simulink model "gm_BlobAnalysisHDL"  (R2022b)
settings: Solver=FixedStepDiscrete  StartTime=0.0  StopTime=1/60  RelTol=1e-3
PreLoadFcn:
  | model_init_cca
InitFcn:
  | model_init_cca
undefined symbols (not defined in the file or in its folder): closenhood, gray, MaxBlobs, numCols, numRows, Rec, rgbmap24, SDTV, Ts
libraries: hdlsllib x37, simulink x21, hdlmdlgenlib x7, visionhdlutilities x5, visionhdlio x2, visiontextngfix x2, visionhdlmorphops x1, visionhdlconversions x1, visionsources x1, visiongeotforms x1
(part 1 of 3)
settings Model: SimulationMode=accelerator  Creator=The MathWorks, Inc.  LastModifiedBy=team06
settings SolverCC: AlgebraicLoopSolver=TrustRegion
settings DataIOCC: SaveOutput=off  SaveTime=off
settings OptimizationCC: BlockReduction=off  ConditionallyExecuteInputs=off  DefaultParameterBehavior=Inlined
settings DebuggingCC: AlgebraicLoopMsg=error  InheritedTsInSrcMsg=none  SingleTaskRateTransMsg=error  ParameterDowncastMsg=none  ParameterOverflowMsg=none  UnconnectedInputMsg=warning  UnconnectedOutputMsg=warning  UnconnectedLineMsg=warning  SFMachineParentedDataDiag=warning
settings HardwareCC: ProdBitPerPointer=32  ProdBitPerSizeT=32  ProdBitPerPtrDiffT=32  ProdLargestAtomicFloat=None  ProdIntDivRoundTo=Undefined  ProdEndianess=Unspecified  ProdWordSize=32  ProdHWDeviceType=ASIC/FPGA->ASIC/FPGA  TargetBitPerPointer=64  TargetBitPerSizeT=64  TargetBitPerPtrDiffT=64  TargetLongLongMode=on  TargetIntDivRoundTo=Zero  TargetEndianess=LittleEndian  TargetWordSize=64  TargetHWDeviceType=Custom Processor->MATLAB Host Computer  ProdEqTarget=off
settings ModelReferenceCC: EnableRefExpFcnMdlSchedulingChecks=on
settings RTWCC: DLArmComputeVersion=19.05

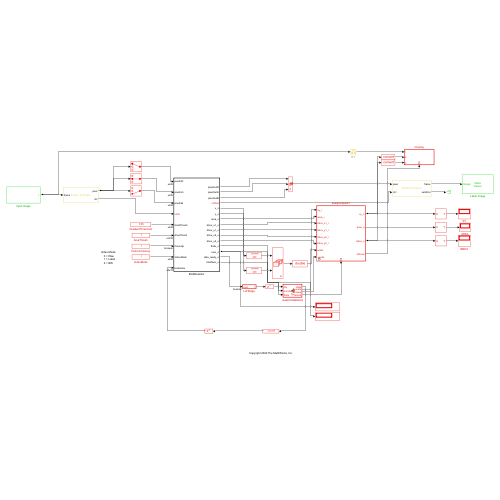
[thumbnail: Simulink's stored preview of the top-level diagram]
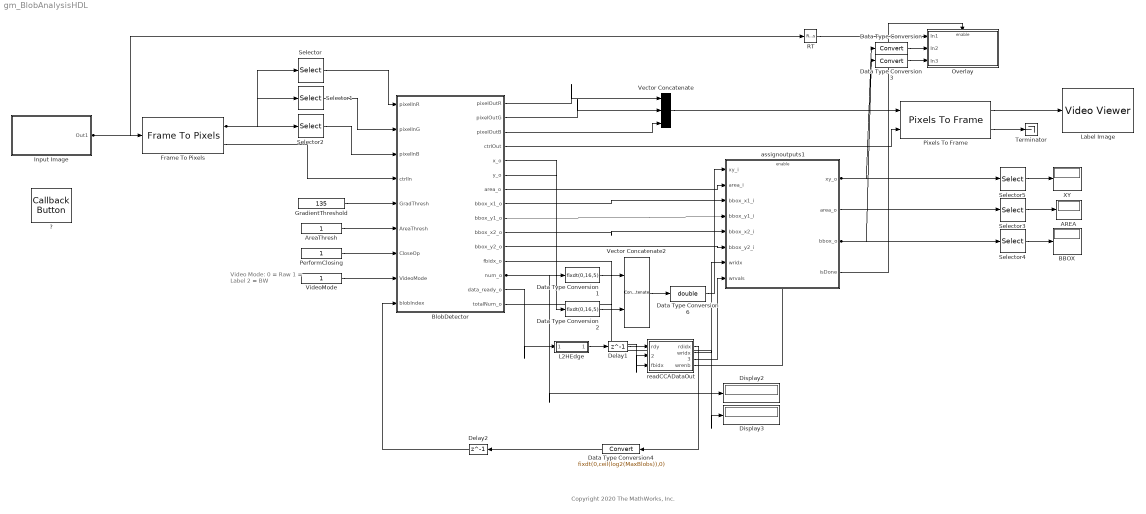
== system gm_BlobAnalysisHDL ==
  note: Copyright 2020 The MathWorks, Inc.
  note: Video Mode:
      |     0 = Raw
      |     1 = Label
      |     2 = BW
  "?" : CallbackButton  ButtonText=?
      settings: ClickFcn=showExample('visionhdl/BlobAnalysisExample')
  AREA : Display
  AreaThresh : Constant  OutDataTypeStr=uint32  SampleTime=-1
  BBOX : Display
  BlobDetector : Subsystem  TreatAsAtomicUnit=on
  Data Type Conversion : DataTypeConversion  SaturateOnIntegerOverflow=off  RndMeth=Floor
  Data Type Conversion1 : DataTypeConversion  OutDataTypeStr=fixdt(0,16,5)  ConvertRealWorld=Stored Integer (SI)  SaturateOnIntegerOverflow=off  RndMeth=Floor
  Data Type Conversion2 : DataTypeConversion  OutDataTypeStr=fixdt(0,16,5)  ConvertRealWorld=Stored Integer (SI)  SaturateOnIntegerOverflow=off  RndMeth=Floor
  Data Type Conversion3 : DataTypeConversion  SaturateOnIntegerOverflow=off  RndMeth=Floor
  Data Type Conversion4 : DataTypeConversion  OutDataTypeStr=fixdt(0,ceil(log2(MaxBlobs)),0)  SaturateOnIntegerOverflow=off  RndMeth=Floor
  Data Type Conversion6 : DataTypeConversion  OutDataTypeStr=double  SaturateOnIntegerOverflow=off  RndMeth=Floor
  Delay1 : Delay  DelayLength=1
  Delay2 : Delay  DelayLength=1
  Display2 : Display
  Display3 : Display
  Frame To Pixels : visionhdlio/Frame To Pixels  NumComponents=3  NumPixels=1  VideoFormat=240p  ActivePixelsPerLine=320  ActiveVideoLines=240  TotalPixelsPerLine=402  TotalVideoLines=324  StartingActiveLine=1  FrontPorch=44  SampleTime=0  VideoFormatCache=240p  ActivePixelsPerLineCache=numCols  ActiveVideoLinesCache=numRows  TotalPixelsPerLineCache=numCols+50  TotalVideoLinesCache=numRows+5  StartingActiveLineCache=2  FrontPorchCache=2
  GradientThreshold : Constant  Value=135  OutDataTypeStr=uint8  SampleTime=-1
  Input Image : Subsystem
  L2HEdge : Subsystem  TreatAsAtomicUnit=on
  Label Image : VideoViewer  FigPos=[539 508 418 304]
  Overlay : Subsystem
  PerformClosing : Constant  OutDataTypeStr=boolean  SampleTime=-1
  Pixels To Frame : visionhdlio/Pixels To Frame  NumComponents=3  NumPixels=1  VideoFormat=240p  ActivePixelsPerLine=320  ActiveVideoLines=240  TotalPixelsPerLine=402  TotalVideoLines=324  VideoFormatCache=240p  ActivePixelsPerLineCache=numCols  ActiveVideoLinesCache=numRows  TotalPixelsPerLineCache=numCols+50  TotalVideoLinesCache=numRows+5
  RT : RateTransition  Deterministic=off  OutPortSampleTimeOpt=Inherit  OutPortSampleTime=1.2796101795549e-07
  Selector : Selector  InputPortWidth=3  IndexOptions=Index vector (dialog)  Indices=1  OutputSizes=1
  Selector1 : Selector  InputPortWidth=3  IndexOptions=Index vector (dialog)  Indices=2  OutputSizes=1
  Selector2 : Selector  InputPortWidth=3  IndexOptions=Index vector (dialog)  Indices=3  OutputSizes=1
  Selector3 : Selector  NumberOfDimensions=2  InputPortWidth=3  IndexOptions=Index vector (dialog),Select all  Indices=1:20,1:200  OutputSizes=1,1
  Selector4 : Selector  NumberOfDimensions=2  InputPortWidth=3  IndexOptions=Index vector (dialog),Select all  Indices=1:20,1:200  OutputSizes=1,1
  Selector5 : Selector  NumberOfDimensions=2  InputPortWidth=3  IndexOptions=Index vector (dialog),Select all  Indices=1:20,1:200  OutputSizes=1,1
  Terminator : Terminator
  Vector Concatenate : Concatenate  NumInputs=3  Mode=Multidimensional array  ConcatenateDimension=2
  Vector Concatenate2 : Concatenate  Mode=Multidimensional array  ConcatenateDimension=2
  VideoMode : Constant  OutDataTypeStr=uint8  SampleTime=-1
  XY : Display
  assignoutputs1 : Subsystem
  readCCADataOut : MATLAB Function  TreatAsAtomicUnit=on  mask{maxnumblobs=MaxBlobs}
      mask prompts: maxnumblobs "Max number of blobs"
  wires:
  Selector5/1 -> XY/1
  Selector4/1 -> BBOX/1
  Selector3/1 -> AREA/1
  Input Image/1(Out1) -> Frame To Pixels/1, RT/1
  Frame To Pixels/1 -> Selector2/1, Selector/1, Selector1/1
  Selector1/1 -> BlobDetector/2(pixelInG)
  readCCADataOut/3(wrvalue) -> assignoutputs1/8(wrvals)
  Data Type Conversion4/1 -> Delay2/1
  Vector Concatenate/1 -> Pixels To Frame/1
  BlobDetector/8(bbox_x1_o) -> assignoutputs1/3(bbox_x1_i)
  RT/1 -> Overlay/1(In1)
  readCCADataOut/2(wridx) -> assignoutputs1/7(wridx)
  L2HEdge/1(Out1) -> Delay1/1
  Vector Concatenate2/1 -> Data Type Conversion6/1
  assignoutputs1/1(xy_o) -> Data Type Conversion/1, Selector5/1
  BlobDetector/10(bbox_x2_o) -> assignoutputs1/5(bbox_x2_i)
  GradientThreshold/1 -> BlobDetector/5(GradThresh)
  Data Type Conversion2/1 -> Vector Concatenate2/2
  Data Type Conversion3/1 -> Overlay/3(In3)
  VideoMode/1 -> BlobDetector/8(VideoMode)
  AreaThresh/1 -> BlobDetector/6(AreaThresh)
  BlobDetector/4(ctrlOut) -> Pixels To Frame/2
  assignoutputs1/4(isDone) -> Overlay/Enable
  Data Type Conversion6/1 -> assignoutputs1/1(xy_i)
  Selector2/1 -> BlobDetector/3(pixelInB)
  PerformClosing/1 -> BlobDetector/7(CloseOp)
  Delay1/1 -> readCCADataOut/1(rdy)
  Frame To Pixels/2 -> BlobDetector/4(ctrlIn)
  BlobDetector/6(y_o) -> Data Type Conversion2/1
  BlobDetector/9(bbox_y1_o) -> assignoutputs1/4(bbox_y1_i)
  BlobDetector/13(num_o) -> Display2/1, readCCADataOut/2(num2rd)
  Pixels To Frame/2 -> Terminator/1
  readCCADataOut/4(wrenb) -> assignoutputs1/Enable
  BlobDetector/12(fbidx_o) -> readCCADataOut/3(fbidx)
  Data Type Conversion1/1 -> Vector Concatenate2/1
  Delay2/1 -> BlobDetector/9(blobIndex)
  Selector/1 -> BlobDetector/1(pixelInR)
  BlobDetector/2(pixelOutG) -> Vector Concatenate/2
  assignoutputs1/2(area_o) -> Selector3/1
  BlobDetector/3(pixelOutB) -> Vector Concatenate/3
  BlobDetector/7(area_o) -> assignoutputs1/2(area_i)
  BlobDetector/11(bbox_y2_o) -> assignoutputs1/6(bbox_y2_i)
  readCCADataOut/1(rdidx) -> Data Type Conversion4/1
  assignoutputs1/3(bbox_o) -> Data Type Conversion3/1, Selector4/1
  BlobDetector/5(x_o) -> Data Type Conversion1/1
  BlobDetector/14(data_ready_o) -> L2HEdge/1(sync)
  Pixels To Frame/1 -> Label Image/1
  Data Type Conversion/1 -> Overlay/2(In2)
  BlobDetector/15(totalNum_o) -> Display3/1
  BlobDetector/1(pixelOutR) -> Vector Concatenate/1

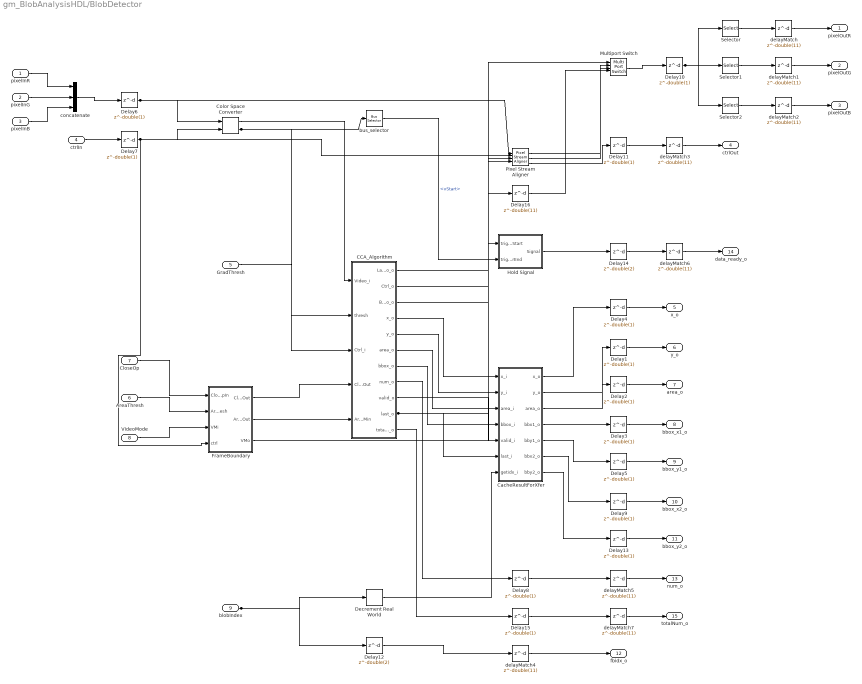
== system gm_BlobAnalysisHDL/BlobDetector ==
  pixelInR : Inport  OutDataTypeStr=uint8  PortDimensions=1  SampleTime=1.2796101795549e-07
  pixelInG : Inport  Port=2  OutDataTypeStr=uint8  PortDimensions=1  SampleTime=1.2796101795549e-07
  pixelInB : Inport  Port=3  OutDataTypeStr=uint8  PortDimensions=1  SampleTime=1.2796101795549e-07
  ctrlIn : Inport  Port=4
  GradThresh : Inport  Port=5  OutDataTypeStr=uint8  PortDimensions=1  SampleTime=1.2796101795549e-07
  AreaThresh : Inport  Port=6  OutDataTypeStr=uint32  PortDimensions=1  SampleTime=1.2796101795549e-07
  CloseOp : Inport  Port=7  OutDataTypeStr=boolean  PortDimensions=1  SampleTime=1.2796101795549e-07
  VideoMode : Inport  Port=8  OutDataTypeStr=uint8  PortDimensions=1  SampleTime=1.2796101795549e-07
  blobIndex : Inport  Port=9  OutDataTypeStr=fixdt(0, 10, 0)  PortDimensions=1  SampleTime=1.2796101795549e-07
  CCA_Algorithm : Subsystem
  CacheResultForXfer : Subsystem
  Color Space Converter : visionhdlconversions/Color Space Converter  Conversion=RGB to intensity  ConversionStandard=Rec. 601 (SDTV)  ScanningStandard=1250/50/2:1  SimulateUsing=Code generation
  Decrement Real World : simulink/Additional Math & Discrete/Additional Math: Increment - Decrement/Decrement Real World
  Delay{1..6,8..10,13,15} (11 alike) : Delay  DelayLength=double(1)  InitialCondition=0  SampleTime=1.2796101795549e-07
  Delay11 : Delay  DelayLength=double(1)  SampleTime=1.2796101795549e-07
  Delay12 : Delay  DelayLength=double(2)  InitialCondition=0  SampleTime=1.2796101795549e-07
  Delay14 : Delay  DelayLength=double(2)  InitialCondition=0  SampleTime=1.2796101795549e-07
  Delay16 : Delay  DelayLength=double(11)  InitialCondition=0  SampleTime=1.2796101795549e-07
  Delay7 : Delay  DelayLength=double(1)  SampleTime=1.2796101795549e-07
  FrameBoundary : Subsystem
  Hold Signal : Subsystem
  Multiport Switch : MultiPortSwitch  DataPortOrder=Zero-based contiguous  DiagnosticForDefault=None  zeroidx=on  OutDataTypeStr=uint8  SampleTime=1.2796101795549e-07  SaturateOnIntegerOverflow=off  InputSameDT=off
  Pixel Stream Aligner : visionhdlutilities/Pixel Stream Aligner  LineBufferSize=2048  MaximumNumberOfLines=size(closenhood.Neighborhood,1)+1  SimulateUsing=Code generation
  Selector : Selector  SampleTime=1.2796101795549e-07  IndexOptions=Index vector (dialog)  Indices=double(1)  OutputSizes=double(1)
  Selector1 : Selector  SampleTime=1.2796101795549e-07  IndexOptions=Index vector (dialog)  Indices=double(2)  OutputSizes=double(1)
  Selector2 : Selector  SampleTime=1.2796101795549e-07  IndexOptions=Index vector (dialog)  Indices=double(3)  OutputSizes=double(1)
  bus_selector : BusSelector  OutputSignals=vStart
  concatenate : Concatenate  NumInputs=3  Mode=Multidimensional array  ConcatenateDimension=2
  delayMatch{,1..7} (8 alike) : Delay  DelayLength=double(11)  InitialCondition=0  SampleTime=1.2796101795549e-07
  pixelOutR : Outport  SampleTime=1.2796101795549e-07  VectorParamsAs1DForOutWhenUnconnected=off
  pixelOutG : Outport  Port=2  SampleTime=1.2796101795549e-07  VectorParamsAs1DForOutWhenUnconnected=off
  pixelOutB : Outport  Port=3  SampleTime=1.2796101795549e-07  VectorParamsAs1DForOutWhenUnconnected=off
  ctrlOut : Outport  Port=4  VectorParamsAs1DForOutWhenUnconnected=off
  x_o : Outport  Port=5  SampleTime=1.2796101795549e-07  VectorParamsAs1DForOutWhenUnconnected=off
  y_o : Outport  Port=6  SampleTime=1.2796101795549e-07  VectorParamsAs1DForOutWhenUnconnected=off
  area_o : Outport  Port=7  SampleTime=1.2796101795549e-07  VectorParamsAs1DForOutWhenUnconnected=off
  bbox_x1_o : Outport  Port=8  SampleTime=1.2796101795549e-07  VectorParamsAs1DForOutWhenUnconnected=off
  bbox_y1_o : Outport  Port=9  SampleTime=1.2796101795549e-07  VectorParamsAs1DForOutWhenUnconnected=off
  bbox_x2_o : Outport  Port=10  SampleTime=1.2796101795549e-07  VectorParamsAs1DForOutWhenUnconnected=off
  bbox_y2_o : Outport  Port=11  SampleTime=1.2796101795549e-07  VectorParamsAs1DForOutWhenUnconnected=off
  fbidx_o : Outport  Port=12  SampleTime=1.2796101795549e-07  VectorParamsAs1DForOutWhenUnconnected=off
  num_o : Outport  Port=13  SampleTime=1.2796101795549e-07  VectorParamsAs1DForOutWhenUnconnected=off
  data_ready_o : Outport  Port=14  SampleTime=1.2796101795549e-07  VectorParamsAs1DForOutWhenUnconnected=off
  totalNum_o : Outport  Port=15  SampleTime=1.2796101795549e-07  VectorParamsAs1DForOutWhenUnconnected=off
  wires:
  pixelInR/1 -> concatenate/1
  pixelInG/1 -> concatenate/2
  pixelInB/1 -> concatenate/3
  ctrlIn/1 -> Delay7/1
  GradThresh/1 -> CCA_Algorithm/2(thresh)
  AreaThresh/1 -> FrameBoundary/2(AreaThresh)
  CloseOp/1 -> FrameBoundary/1(CloseOpIn)
  VideoMode/1 -> FrameBoundary/3(VMi)
  blobIndex/1 -> Decrement Real World/1, Delay12/1
  bus_selector/1 -> Hold Signal/2(triggerEnd)  "<vStart>"
  CCA_Algorithm/1(LabelVideo_o) -> Pixel Stream Aligner/3
  CCA_Algorithm/2(Ctrl_o) -> Pixel Stream Aligner/4
  CCA_Algorithm/3(BWVideo_o) -> Delay16/1
  CCA_Algorithm/4(x_o) -> CacheResultForXfer/1(x_i)
  CCA_Algorithm/5(y_o) -> CacheResultForXfer/2(y_i)
  CCA_Algorithm/6(area_o) -> CacheResultForXfer/3(area_i)
  CCA_Algorithm/7(bbox_o) -> CacheResultForXfer/4(bbox_i)
  CCA_Algorithm/8(num_o) -> Delay8/1
  CCA_Algorithm/9(valid_o) -> CacheResultForXfer/5(valid_i)
  CCA_Algorithm/10(last_o) -> Hold Signal/1(triggerStart), CacheResultForXfer/6(last_i)
  CCA_Algorithm/11(totalNum_o) -> Delay15/1
  CacheResultForXfer/1(x_o) -> Delay4/1
  CacheResultForXfer/2(y_o) -> Delay1/1
  CacheResultForXfer/3(area_o) -> Delay2/1
  CacheResultForXfer/4(bbx1_o) -> Delay3/1
  CacheResultForXfer/5(bby1_o) -> Delay5/1
  CacheResultForXfer/6(bbx2_o) -> Delay9/1
  CacheResultForXfer/7(bby2_o) -> Delay13/1
  Color Space Converter/1 -> CCA_Algorithm/1(Video_i)
  Color Space Converter/2 -> bus_selector/1, CCA_Algorithm/3(Ctrl_i)
  Decrement Real World/1 -> CacheResultForXfer/7(getidx_i)
  Delay1/1 -> y_o/1
  Delay10/1 -> Selector2/1, Selector1/1, Selector/1
  delayMatch3/1 -> ctrlOut/1
  delayMatch4/1 -> fbidx_o/1
  Delay13/1 -> bbox_y2_o/1
  delayMatch6/1 -> data_ready_o/1
  delayMatch7/1 -> totalNum_o/1
  Delay16/1 -> Multiport Switch/4
  Delay2/1 -> area_o/1
  Delay3/1 -> bbox_x1_o/1
  Delay4/1 -> x_o/1
  Delay5/1 -> bbox_y1_o/1
  Delay6/1 -> Pixel Stream Aligner/1, Color Space Converter/1
  Delay7/1 -> FrameBoundary/4(ctrl), Pixel Stream Aligner/2, Color Space Converter/2
  delayMatch5/1 -> num_o/1
  Delay9/1 -> bbox_x2_o/1
  FrameBoundary/1(CloseOpOut) -> CCA_Algorithm/4(CloseOpOut)
  FrameBoundary/2(AreaThreshOut) -> CCA_Algorithm/5(AreaMin)
  FrameBoundary/3(VMo) -> Multiport Switch/1
  Hold Signal/1(Signal) -> Delay14/1
  Multiport Switch/1 -> Delay10/1
  Pixel Stream Aligner/1 -> Multiport Switch/2
  Pixel Stream Aligner/2 -> Multiport Switch/3
  Pixel Stream Aligner/3 -> Delay11/1
  delayMatch/1 -> pixelOutR/1
  delayMatch1/1 -> pixelOutG/1
  delayMatch2/1 -> pixelOutB/1
  concatenate/1 -> Delay6/1
  Selector/1 -> delayMatch/1
  Selector1/1 -> delayMatch1/1
  Selector2/1 -> delayMatch2/1
  Delay11/1 -> delayMatch3/1
  Delay12/1 -> delayMatch4/1
  Delay8/1 -> delayMatch5/1
  Delay14/1 -> delayMatch6/1
  Delay15/1 -> delayMatch7/1

== system gm_BlobAnalysisHDL/Input Image ==
  Constant : Constant  Value=true  VectorParams1D=off  SampleTime=-1
  Data Type Conversion : DataTypeConversion  OutDataTypeStr=uint8  SaturateOnIntegerOverflow=off  RndMeth=Floor
  Delay : Delay  DelayLength=1  InitialCondition=0  UseCircularBuffer=on
  Delay1 : Delay  DelayLength=1  InitialCondition=0  ShowEnablePort=on  UseCircularBuffer=on
      settings: InputPortMap=u0,e6
  Image From File : visionsources/Image From File  Tag=vipblks_nd  FileName=coins.png  Ts=1/60  imagePorts=One multidimensional signal  OutPortLabels=R|G|B  ImageDataType=Inherit from input image  sdImageDataType=uint(8)  Signed=on  WordLength=16  FractionLengthMode=User-defined  FractionLength=15
  Matrix Concatenate : Concatenate  NumInputs=3  Mode=Multidimensional array  ConcatenateDimension=3
  Matrix Concatenate1 : Concatenate  Mode=Multidimensional array  ConcatenateDimension=2
  Multiport Switch : MultiPortSwitch  DataPortOrder=Zero-based contiguous  Inputs=2  zeroidx=on  SaturateOnIntegerOverflow=off  InputSameDT=off
  Resize : visiongeotforms/Resize  specify=Number of output rows and columns  rfactor=[200 150]  outCols=25  outRows=25  outRowsCols=[240 320]  interp_method=Bilinear  antialias=on  useROI=off  roiFlag=off  roundingMode=Nearest  overflowMode=on  prodOutputMode=Binary point scaling  prodOutputWordLength=32  prodOutputFracLength=10
  Selector : Selector  NumberOfDimensions=2  InputPortWidth=3  IndexOptions=Select all,Index vector (dialog)  Indices=[1 3],301:320  OutputSizes=1,1
  Selector1 : Selector  NumberOfDimensions=2  InputPortWidth=3  IndexOptions=Select all,Index vector (dialog)  Indices=[1 3],1:300  OutputSizes=1,1
  Out1 : Outport
  wires:
  Data Type Conversion/1 -> Out1/1
  Delay1/1 -> Multiport Switch/1
  Constant/1 -> Delay1/1, Delay1/2
  Delay/1 -> Multiport Switch/3
  Selector1/1 -> Matrix Concatenate1/2
  Selector/1 -> Matrix Concatenate1/1
  Multiport Switch/1 -> Selector/1, Selector1/1, Matrix Concatenate/1, Matrix Concatenate/2, Matrix Concatenate/3
  Matrix Concatenate1/1 -> Delay/1
  Resize/1 -> Multiport Switch/2
  Image From File/1 -> Resize/1
  Matrix Concatenate/1 -> Data Type Conversion/1

== system gm_BlobAnalysisHDL/L2HEdge ==
  sync : Inport  OutDataTypeStr=boolean
  Logical Operator : Logic  Operator=XOR  IconShape=distinctive  AllPortsSameDT=off  OutDataTypeStr=boolean
  Logical Operator2 : Logic  IconShape=distinctive  AllPortsSameDT=off  OutDataTypeStr=boolean
  Unit Delay : UnitDelay  SampleTime=-1  HasFrameUpgradeWarning=on
  Out1 : Outport  VectorParamsAs1DForOutWhenUnconnected=off
  wires:
  Logical Operator2/1 -> Out1/1
  Logical Operator/1 -> Logical Operator2/1
  Unit Delay/1 -> Logical Operator/1
  sync/1 -> Logical Operator2/2, Logical Operator/2, Unit Delay/1

== system gm_BlobAnalysisHDL/Overlay ==
  In1 : Inport
  In2 : Inport  Port=2
  In3 : Inport  Port=3
  Enable : EnablePort
  Draw Markers : visiontextngfix/Draw Markers  shape=Plus  size=1  fill=on  fillClrSource=Specify via dialog  display=User-specified value  intensity=200  color=[255 20 20]  opacity=1  viewport=Entire image  antialiasing=off  inType=Obsolete  imagePorts=One multidimensional signal  roundingMode=Floor  overflowMode=off  memoryMode=Specify word length  memoryWordLength=16  memoryFracLength=15  prodOutputMode=Binary point scaling  prodOutputWordLength=32  prodOutputFracLength=14
  Draw Shapes : visiontextngfix/Draw Shapes  shape=Rectangles  fill=off  lineWidth=1  fillClrSource=Specify via dialog  display=User-specified value  intensity=200  color=[20 255 10]  opacity=0.6  viewport=Entire image  antialiasing=off  inType=Obsolete  imagePorts=One multidimensional signal  roundingMode=Floor  overflowMode=off  memoryMode=Specify word length  memoryWordLength=16  prodOutputMode=Binary point scaling  prodOutputWordLength=32  prodOutputFracLength=14  memoryFracLength=15
  Results On Image : VideoViewer  colormapValue=gray(256)  FigPos=[117 509 417 304]
  wires:
  Draw Markers/1 -> Draw Shapes/1
  In3/1 -> Draw Shapes/2
  In2/1 -> Draw Markers/2
  In1/1 -> Draw Markers/1
  Draw Shapes/1 -> Results On Image/1

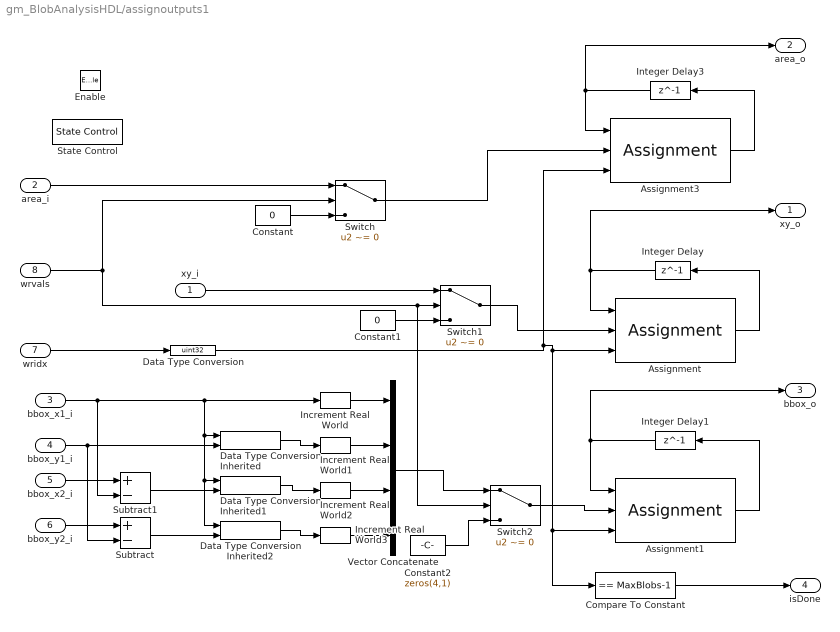
== system gm_BlobAnalysisHDL/assignoutputs1 ==
  xy_i : Inport
  area_i : Inport  Port=2
  bbox_x1_i : Inport  Port=3
  bbox_y1_i : Inport  Port=4
  bbox_x2_i : Inport  Port=5
  bbox_y2_i : Inport  Port=6
  wridx : Inport  Port=7
  wrvals : Inport  Port=8
  Enable : EnablePort
  Assignment : Assignment  NumberOfDimensions=2  DiagnosticForDimensions=Warning  IndexOptions=Starting index (port),Assign all  Indices=1,1  OutputSizes=1,1
  Assignment1 : Assignment  NumberOfDimensions=2  DiagnosticForDimensions=Warning  IndexOptions=Starting index (port),Assign all  Indices=1,1  OutputSizes=1,1
  Assignment3 : Assignment  NumberOfDimensions=2  DiagnosticForDimensions=Warning  IndexOptions=Starting index (port),Assign all  Indices=1,1  OutputSizes=1,1
  Compare To Constant : simulink/Logic and Bit Operations/Compare To Constant  relop===  const=MaxBlobs-1  OutDataTypeStr=boolean
  Constant : Constant  Value=0  OutDataTypeStr=Inherit: Inherit via back propagation  SampleTime=-1
  Constant1 : Constant  Value=0  OutDataTypeStr=Inherit: Inherit via back propagation  SampleTime=-1
  Constant2 : Constant  Value=zeros(4,1)  OutDataTypeStr=Inherit: Inherit via back propagation  SampleTime=-1
  Data Type Conversion Inherited : simulink/Signal Attributes/Data Type Conversion Inherited  ConvertRealWorld=Real World Value  DoSatur=off
  Data Type Conversion Inherited1 : simulink/Signal Attributes/Data Type Conversion Inherited  ConvertRealWorld=Real World Value  DoSatur=off
  Data Type Conversion Inherited2 : simulink/Signal Attributes/Data Type Conversion Inherited  ConvertRealWorld=Real World Value  DoSatur=off
  Data Type Conversion : DataTypeConversion  OutDataTypeStr=uint32  SaturateOnIntegerOverflow=off  RndMeth=Floor
  Increment Real World{,1..3} (4 alike) : simulink/Additional Math & Discrete/Additional Math: Increment - Decrement/Increment Real World
  Integer Delay : Delay  DelayLength=1  InitialCondition=zeros(MaxBlobs,2)
  Integer Delay1 : Delay  DelayLength=1  InitialCondition=zeros(MaxBlobs,4)
  Integer Delay3 : Delay  DelayLength=1  InitialCondition=zeros(MaxBlobs,1)
  State Control : StateControl  StateControl=Synchronous
  Subtract : Sum  Inputs=+-  OutDataTypeStr=Inherit: Same as first input
  Subtract1 : Sum  Inputs=+-  OutDataTypeStr=Inherit: Same as first input
  Switch : Switch  Criteria=u2 ~= 0  SaturateOnIntegerOverflow=off  InputSameDT=off
  Switch1 : Switch  Criteria=u2 ~= 0  SaturateOnIntegerOverflow=off  InputSameDT=off
  Switch2 : Switch  Criteria=u2 ~= 0  SaturateOnIntegerOverflow=off  InputSameDT=off
  Vector Concatenate : Concatenate  NumInputs=4  Mode=Multidimensional array  ConcatenateDimension=2
  xy_o : Outport  VectorParamsAs1DForOutWhenUnconnected=off
  area_o : Outport  Port=2  VectorParamsAs1DForOutWhenUnconnected=off
  bbox_o : Outport  Port=3  VectorParamsAs1DForOutWhenUnconnected=off
  isDone : Outport  Port=4  VectorParamsAs1DForOutWhenUnconnected=off
  wires:
  wridx/1 -> Data Type Conversion/1
  Compare To Constant/1 -> isDone/1
  Data Type Conversion/1 -> Assignment1/3, Compare To Constant/1, Assignment/3, Assignment3/3
  Switch2/1 -> Assignment1/2
  Constant2/1 -> Switch2/3
  xy_i/1 -> Switch1/1
  Constant1/1 -> Switch1/3
  Switch/1 -> Assignment3/2
  Constant/1 -> Switch/3
  area_i/1 -> Switch/1
  wrvals/1 -> Switch/2, Switch1/2, Switch2/2
  Assignment/1 -> Integer Delay/1
  Switch1/1 -> Assignment/2
  Integer Delay/1 -> Assignment/1, xy_o/1
  Integer Delay1/1 -> bbox_o/1, Assignment1/1
  Assignment1/1 -> Integer Delay1/1
  Vector Concatenate/1 -> Switch2/1
  bbox_x1_i/1 -> Data Type Conversion Inherited2/1, Data Type Conversion Inherited1/1, Data Type Conversion Inherited/1, Increment Real World/1, Subtract1/2
  bbox_y1_i/1 -> Data Type Conversion Inherited/2, Subtract/2
  Increment Real World/1 -> Vector Concatenate/1
  Increment Real World1/1 -> Vector Concatenate/2
  bbox_x2_i/1 -> Subtract1/1
  bbox_y2_i/1 -> Subtract/1
  Increment Real World2/1 -> Vector Concatenate/3
  Increment Real World3/1 -> Vector Concatenate/4
  Assignment3/1 -> Integer Delay3/1
  Integer Delay3/1 -> Assignment3/1, area_o/1
  Data Type Conversion Inherited/1 -> Increment Real World1/1
  Subtract1/1 -> Data Type Conversion Inherited1/2
  Subtract/1 -> Data Type Conversion Inherited2/2
  Data Type Conversion Inherited1/1 -> Increment Real World2/1
  Data Type Conversion Inherited2/1 -> Increment Real World3/1

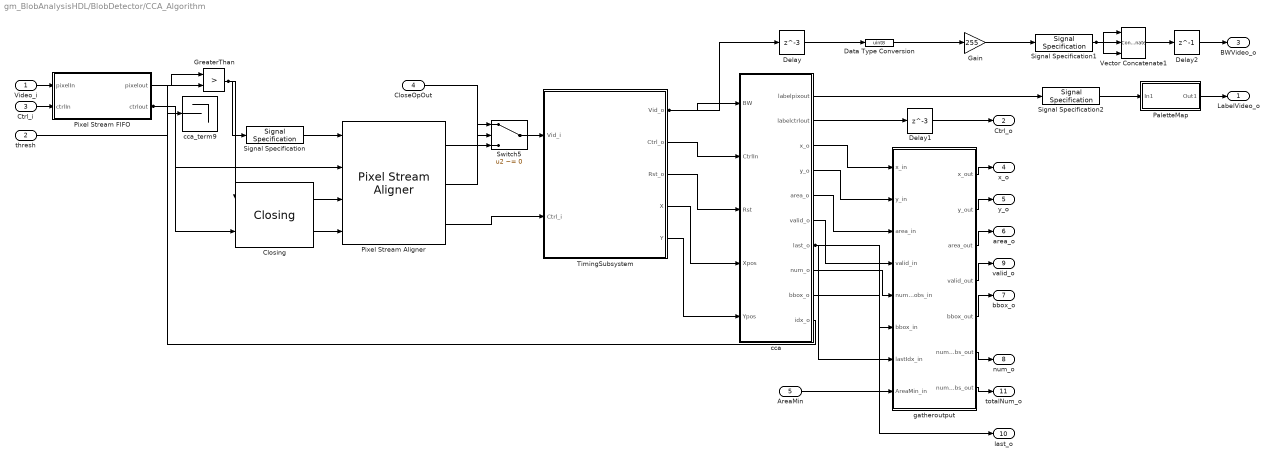
== system gm_BlobAnalysisHDL/BlobDetector/CCA_Algorithm ==
  Video_i : Inport  OutDataTypeStr=uint8  PortDimensions=1  SampleTime=1.2796101795549e-07
  thresh : Inport  Port=2  OutDataTypeStr=uint8  PortDimensions=1  SampleTime=1.2796101795549e-07
  Ctrl_i : Inport  Port=3
  CloseOpOut : Inport  Port=4  OutDataTypeStr=boolean  PortDimensions=1  SampleTime=1.2796101795549e-07
  AreaMin : Inport  Port=5  OutDataTypeStr=uint32  PortDimensions=1  SampleTime=1.2796101795549e-07
  Closing : visionhdlmorphops/Closing  Neighborhood=closenhood.Neighborhood  LineBufferSize=2048  PaddingMethod=Constant  SimulateUsing=Code generation
  Data Type Conversion : DataTypeConversion  OutDataTypeStr=uint8  SaturateOnIntegerOverflow=off  RndMeth=Floor
  Delay : Delay  DelayLength=3
  Delay1 : Delay  DelayLength=3
  Delay2 : Delay  DelayLength=1
  Gain : Gain  Gain=255  OutDataTypeStr=uint8
  GreaterThan : RelationalOperator  Operator=>  OutDataTypeStr=boolean  RndMeth=Simplest  InputSameDT=off
  PaletteMap : Subsystem
  Pixel Stream Aligner : visionhdlutilities/Pixel Stream Aligner  LineBufferSize=2048  MaximumNumberOfLines=size(closenhood.Neighborhood,1)+1  SimulateUsing=Code generation
  Pixel Stream FIFO : Subsystem  mask(Pixel Stream FIFO){LineBufferSize=double(2048)}
      mask prompts: LineBufferSize "Line buffer size"
      mask help: Buffer bursts of pixels into a contiguous stream
      mask init:
      | LineBufferSize = double(2048);
      | addrBits = double(11);
      mask Display:
      | disp('Pixel Stream FIFO');
      | port_label('input',1,'pixel');
      | port_label('input',2,'ctrl');
      | port_label('output',1,'pixel');
      | port_label('output',2,'ctrl');
  Signal Specification : SignalSpecification  Dimensions=1
  Signal Specification1 : SignalSpecification  Dimensions=1
  Signal Specification2 : SignalSpecification  Dimensions=1
  Switch5 : Switch  Criteria=u2 ~= 0  SaturateOnIntegerOverflow=off  InputSameDT=off
  TimingSubsystem : Subsystem
  Vector Concatenate1 : Concatenate  NumInputs=3  Mode=Multidimensional array  ConcatenateDimension=2
  cca : Subsystem  mask{MaxBlobs=double(1024)}
      mask prompts: MaxBlobs "Max Blobs"
  cca_term9 : Terminator
  gatheroutput : Subsystem
  LabelVideo_o : Outport  SampleTime=1.2796101795549e-07  VectorParamsAs1DForOutWhenUnconnected=off
  Ctrl_o : Outport  Port=2  VectorParamsAs1DForOutWhenUnconnected=off
  BWVideo_o : Outport  Port=3  SampleTime=1.2796101795549e-07  VectorParamsAs1DForOutWhenUnconnected=off
  x_o : Outport  Port=4  SampleTime=1.2796101795549e-07  VectorParamsAs1DForOutWhenUnconnected=off
  y_o : Outport  Port=5  SampleTime=1.2796101795549e-07  VectorParamsAs1DForOutWhenUnconnected=off
  area_o : Outport  Port=6  SampleTime=1.2796101795549e-07  VectorParamsAs1DForOutWhenUnconnected=off
  bbox_o : Outport  Port=7  SampleTime=1.2796101795549e-07  VectorParamsAs1DForOutWhenUnconnected=off
  num_o : Outport  Port=8  SampleTime=1.2796101795549e-07  VectorParamsAs1DForOutWhenUnconnected=off
  valid_o : Outport  Port=9  SampleTime=1.2796101795549e-07  VectorParamsAs1DForOutWhenUnconnected=off
  last_o : Outport  Port=10  SampleTime=1.2796101795549e-07  VectorParamsAs1DForOutWhenUnconnected=off
  totalNum_o : Outport  Port=11  SampleTime=1.2796101795549e-07  VectorParamsAs1DForOutWhenUnconnected=off
  wires:
  Closing/1 -> Pixel Stream Aligner/3
  Closing/2 -> Pixel Stream Aligner/4
  Data Type Conversion/1 -> Gain/1
  Delay/1 -> Data Type Conversion/1
  Delay1/1 -> Ctrl_o/1
  Delay2/1 -> BWVideo_o/1
  Gain/1 -> Signal Specification1/1
  GreaterThan/1 -> Signal Specification/1, Closing/1
  PaletteMap/1(Out1) -> LabelVideo_o/1
  Pixel Stream Aligner/1 -> Switch5/3
  Pixel Stream Aligner/2 -> Switch5/1
  Pixel Stream Aligner/3 -> TimingSubsystem/2(Ctrl_i)
  Pixel Stream FIFO/1(pixelout) -> GreaterThan/1
  Pixel Stream FIFO/2(ctrlout) -> Pixel Stream Aligner/2, Closing/2
  Signal Specification/1 -> Pixel Stream Aligner/1
  Signal Specification1/1 -> Vector Concatenate1/3, Vector Concatenate1/2, Vector Concatenate1/1
  Signal Specification2/1 -> PaletteMap/1(In1)
  Switch5/1 -> TimingSubsystem/1(Vid_i)
  TimingSubsystem/1(Vid_o) -> Delay/1, cca/1(BW)
  TimingSubsystem/2(Ctrl_o) -> cca/2(CtrlIn)
  TimingSubsystem/3(Rst_o) -> cca/3(Rst)
  TimingSubsystem/4(X) -> cca/4(Xpos)
  TimingSubsystem/5(Y) -> cca/5(Ypos)
  Vector Concatenate1/1 -> Delay2/1
  cca/1(labelpixout) -> Signal Specification2/1
  cca/2(labelctrlout) -> Delay1/1
  cca/3(x_o) -> gatheroutput/1(x_in)
  cca/4(y_o) -> gatheroutput/2(y_in)
  cca/5(area_o) -> gatheroutput/3(area_in)
  cca/6(valid_o) -> gatheroutput/4(valid_in)
  cca/7(last_o) -> gatheroutput/7(lastIdx_in), last_o/1
  cca/8(num_o) -> gatheroutput/5(numTotalBlobs_in)
  cca/9(bbox_o) -> gatheroutput/6(bbox_in)
  cca/10(idx_o) -> cca_term9/1
  gatheroutput/1(x_out) -> x_o/1
  gatheroutput/2(y_out) -> y_o/1
  gatheroutput/3(area_out) -> area_o/1
  gatheroutput/4(valid_out) -> valid_o/1
  gatheroutput/5(bbox_out) -> bbox_o/1
  gatheroutput/6(numBlobs_out) -> num_o/1
  gatheroutput/7(numTotalBlobs_out) -> totalNum_o/1
  Video_i/1 -> Pixel Stream FIFO/1(pixelIn)
  thresh/1 -> GreaterThan/2
  Ctrl_i/1 -> Pixel Stream FIFO/2(ctrlIn)
  CloseOpOut/1 -> Switch5/2
  AreaMin/1 -> gatheroutput/8(AreaMin_in)

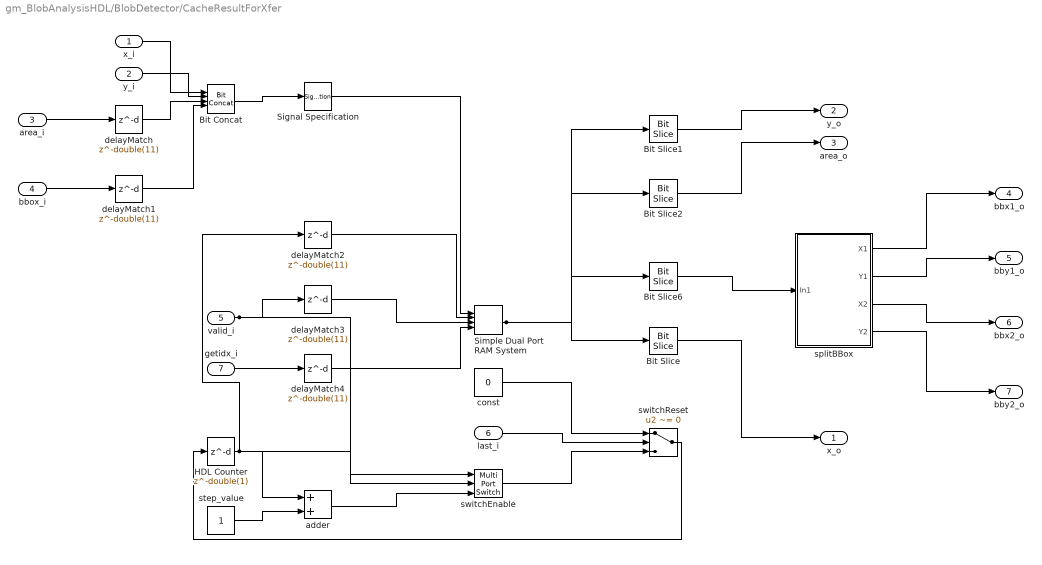
== system gm_BlobAnalysisHDL/BlobDetector/CacheResultForXfer ==
  x_i : Inport  OutDataTypeStr=fixdt(0, 16, 5)  PortDimensions=1  SampleTime=1.2796101795549e-07
  y_i : Inport  Port=2  OutDataTypeStr=fixdt(0, 16, 5)  PortDimensions=1  SampleTime=1.2796101795549e-07
  area_i : Inport  Port=3  OutDataTypeStr=fixdt(0, 17, 0)  PortDimensions=1  SampleTime=1.2796101795549e-07
  bbox_i : Inport  Port=4  OutDataTypeStr=fixdt(0, 34, 0)  PortDimensions=1  SampleTime=1.2796101795549e-07
  valid_i : Inport  Port=5  OutDataTypeStr=boolean  PortDimensions=1  SampleTime=1.2796101795549e-07
  last_i : Inport  Port=6  OutDataTypeStr=boolean  PortDimensions=1  SampleTime=1.2796101795549e-07
  getidx_i : Inport  Port=7  OutDataTypeStr=fixdt(0, 10, 0)  PortDimensions=1  SampleTime=1.2796101795549e-07
  Bit Concat : hdlsllib/Logic and Bit Operations/Bit Concat  numInputs=4
  Bit Slice : hdlsllib/Logic and Bit Operations/Bit Slice  lidx=double(82)  ridx=double(67)
  Bit Slice1 : hdlsllib/Logic and Bit Operations/Bit Slice  lidx=double(66)  ridx=double(51)
  Bit Slice2 : hdlsllib/Logic and Bit Operations/Bit Slice  lidx=double(50)  ridx=double(34)
  Bit Slice6 : hdlsllib/Logic and Bit Operations/Bit Slice  lidx=double(33)  ridx=double(0)
  HDL Counter : Delay  DelayLength=double(1)  InitialCondition=0  SampleTime=1.2796101795549e-07
  Signal Specification : SignalSpecification  OutDataTypeStr=fixdt(0, 83, 0)  Dimensions=1
  Simple Dual Port RAM System : hdlsllib/HDL RAMs/Simple Dual Port RAM System  RAMType=Simple dual port  WriteOutputValue=New data  RAMInitialValue=fi(0,0,107,0)  SimulateUsing=Code generation
  adder : Sum  AccumDataTypeStr=fixdt(0, 10, 0)  OutDataTypeStr=fixdt(0, 10, 0)  SampleTime=1.2796101795549e-07
  const : Constant  Value=0  VectorParams1D=off  OutDataTypeStr=fixdt(0, 10, 0)  SampleTime=1.2796101795549e-07
  delayMatch{,1..4} (5 alike) : Delay  DelayLength=double(11)  InitialCondition=0  SampleTime=1.2796101795549e-07
  splitBBox : Subsystem
  step_value : Constant  VectorParams1D=off  OutDataTypeStr=fixdt(0, 10, 0)  SampleTime=1.2796101795549e-07
  switchEnable : MultiPortSwitch  DataPortOrder=Zero-based contiguous  Inputs=2  DiagnosticForDefault=None  zeroidx=on  OutDataTypeStr=fixdt(0, 10, 0)  SampleTime=1.2796101795549e-07  SaturateOnIntegerOverflow=off  InputSameDT=off
  switchReset : Switch  Criteria=u2 ~= 0  Threshold=double(0)  OutDataTypeStr=fixdt(0, 10, 0)  SampleTime=1.2796101795549e-07  SaturateOnIntegerOverflow=off  InputSameDT=off
  x_o : Outport  SampleTime=1.2796101795549e-07  VectorParamsAs1DForOutWhenUnconnected=off
  y_o : Outport  Port=2  SampleTime=1.2796101795549e-07  VectorParamsAs1DForOutWhenUnconnected=off
  area_o : Outport  Port=3  SampleTime=1.2796101795549e-07  VectorParamsAs1DForOutWhenUnconnected=off
  bbx1_o : Outport  Port=4  SampleTime=1.2796101795549e-07  VectorParamsAs1DForOutWhenUnconnected=off
  bby1_o : Outport  Port=5  SampleTime=1.2796101795549e-07  VectorParamsAs1DForOutWhenUnconnected=off
  bbx2_o : Outport  Port=6  SampleTime=1.2796101795549e-07  VectorParamsAs1DForOutWhenUnconnected=off
  bby2_o : Outport  Port=7  SampleTime=1.2796101795549e-07  VectorParamsAs1DForOutWhenUnconnected=off
  wires:
  delayMatch/1 -> Bit Concat/3
  delayMatch1/1 -> Bit Concat/4
  delayMatch3/1 -> Simple Dual Port RAM System/3
  delayMatch4/1 -> Simple Dual Port RAM System/4
  Bit Concat/1 -> Signal Specification/1
  Bit Slice/1 -> x_o/1
  Bit Slice1/1 -> y_o/1
  Bit Slice2/1 -> area_o/1
  Bit Slice6/1 -> splitBBox/1(In1)
  Signal Specification/1 -> Simple Dual Port RAM System/1
  Simple Dual Port RAM System/1 -> Bit Slice6/1, Bit Slice2/1, Bit Slice1/1, Bit Slice/1
  splitBBox/1(X1) -> bbx1_o/1
  splitBBox/2(Y1) -> bby1_o/1
  splitBBox/3(X2) -> bbx2_o/1
  splitBBox/4(Y2) -> bby2_o/1
  delayMatch2/1 -> Simple Dual Port RAM System/2
  const/1 -> switchReset/1
  step_value/1 -> adder/2
  x_i/1 -> Bit Concat/1
  y_i/1 -> Bit Concat/2
  area_i/1 -> delayMatch/1
  bbox_i/1 -> delayMatch1/1
  valid_i/1 -> delayMatch3/1, switchEnable/1
  last_i/1 -> switchReset/2
  getidx_i/1 -> delayMatch4/1
  HDL Counter/1 -> delayMatch2/1, switchEnable/2, adder/1
  adder/1 -> switchEnable/3
  switchEnable/1 -> switchReset/3
  switchReset/1 -> HDL Counter/1

== system gm_BlobAnalysisHDL/BlobDetector/FrameBoundary ==
  CloseOpIn : Inport  OutDataTypeStr=boolean  PortDimensions=1  SampleTime=1.2796101795549e-07
  AreaThresh : Inport  Port=2  OutDataTypeStr=uint32  PortDimensions=1  SampleTime=1.2796101795549e-07
  VMi : Inport  Port=3  OutDataTypeStr=uint8  PortDimensions=1  SampleTime=1.2796101795549e-07
  ctrl : Inport  Port=4
  Delay2_lowered : Delay  DelayLength=double(1)  InitialCondition=0  SampleTime=1.2796101795549e-07
  Delay3_lowered : Delay  DelayLength=double(1)  InitialCondition=0  SampleTime=1.2796101795549e-07
  Delay_Switch : Switch  Criteria=u2 ~= 0  Threshold=double(0)  OutDataTypeStr=boolean  SampleTime=1.2796101795549e-07  SaturateOnIntegerOverflow=off  InputSameDT=off
  Delay_Switch1 : Switch  Criteria=u2 ~= 0  Threshold=double(0)  OutDataTypeStr=uint32  SampleTime=1.2796101795549e-07  SaturateOnIntegerOverflow=off  InputSameDT=off
  Delay_Switch2 : Switch  Criteria=u2 ~= 0  Threshold=double(0)  OutDataTypeStr=uint8  SampleTime=1.2796101795549e-07  SaturateOnIntegerOverflow=off  InputSameDT=off
  Delay_lowered : Delay  DelayLength=double(1)  InitialCondition=0  SampleTime=1.2796101795549e-07
  Logical Operator : Logic  AllPortsSameDT=off  OutDataTypeStr=boolean  SampleTime=1.2796101795549e-07
  StateControl : StateControl  StateControl=Synchronous
  bus_selector : BusSelector  OutputSignals=vStart,valid
  CloseOpOut : Outport  SampleTime=1.2796101795549e-07  VectorParamsAs1DForOutWhenUnconnected=off
  AreaThreshOut : Outport  Port=2  SampleTime=1.2796101795549e-07  VectorParamsAs1DForOutWhenUnconnected=off
  VMo : Outport  Port=3  SampleTime=1.2796101795549e-07  VectorParamsAs1DForOutWhenUnconnected=off
  wires:
  Delay_lowered/1 -> CloseOpOut/1, Delay_Switch/3
  Delay2_lowered/1 -> AreaThreshOut/1, Delay_Switch1/3
  Delay3_lowered/1 -> VMo/1, Delay_Switch2/3
  Logical Operator/1 -> Delay_Switch/2, Delay_Switch1/2, Delay_Switch2/2
  bus_selector/1 -> Logical Operator/1  "<vStart>"
  bus_selector/2 -> Logical Operator/2  "<valid>"
  CloseOpIn/1 -> Delay_Switch/1
  AreaThresh/1 -> Delay_Switch1/1
  VMi/1 -> Delay_Switch2/1
  ctrl/1 -> bus_selector/1
  Delay_Switch/1 -> Delay_lowered/1
  Delay_Switch1/1 -> Delay2_lowered/1
  Delay_Switch2/1 -> Delay3_lowered/1

== system gm_BlobAnalysisHDL/BlobDetector/Hold Signal ==
  triggerStart : Inport  OutDataTypeStr=boolean  PortDimensions=1  SampleTime=1.2796101795549e-07
  triggerEnd : Inport  Port=2  OutDataTypeStr=boolean  PortDimensions=1  SampleTime=1.2796101795549e-07
  Constant5 : Constant  Value=0  OutDataTypeStr=boolean  SampleTime=-1
  Constant6 : Constant  OutDataTypeStr=boolean  SampleTime=-1
  Delay6 : Delay  DelayLength=1  InitialCondition=0  UseCircularBuffer=on
  Logical Operator : Logic  IconShape=distinctive  AllPortsSameDT=off  OutDataTypeStr=boolean
  Logical Operator1 : Logic  Operator=NOT  IconShape=distinctive  AllPortsSameDT=off  OutDataTypeStr=boolean
  Switch3 : Switch  Criteria=u2 ~= 0  SaturateOnIntegerOverflow=off  InputSameDT=off
  Switch4 : Switch  Criteria=u2 ~= 0  SaturateOnIntegerOverflow=off  InputSameDT=off
  Signal : Outport  SampleTime=1.2796101795549e-07  VectorParamsAs1DForOutWhenUnconnected=off
  wires:
  Constant5/1 -> Switch3/1
  Constant6/1 -> Switch4/1
  Logical Operator/1 -> Switch3/2
  Logical Operator1/1 -> Logical Operator/2
  Switch3/1 -> Signal/1, Delay6/1
  triggerStart/1 -> Logical Operator1/1, Switch4/2
  triggerEnd/1 -> Logical Operator/1
  Switch4/1 -> Switch3/3
  Delay6/1 -> Switch4/3

== system gm_BlobAnalysisHDL/BlobDetector/CCA_Algorithm/PaletteMap ==
  In1 : Inport  OutDataTypeStr=fixdt(0, 10, 0)  PortDimensions=1  SampleTime=1.2796101795549e-07
  1-D Lookup Table : Lookup_n-D  NumberOfTableDimensions=1  LookupTableObject=''  BreakpointsSpecification=Even spacing  BreakpointsForDimension1=[-5:5]  BreakpointsForDimension1FirstPoint=0  IndexSearchMethod=Evenly spaced points  Table=rgbmap24  TableDataTypeStr=Inherit: Inherit from 'Table data'  InterpMethod=Flat  DiagnosticForOutOfRangeInput=Error  InternalRulePriority=Speed  OutDataTypeStr=Inherit: Inherit from 'Table data'  RndMeth=Simplest
  Add : Sum
  Constant : Constant  Value=uint8(1)  SampleTime=-1
  Delay : Delay  DelayLength=1
  Gain1 : Gain  Gain=256/(2^ceil(log2(MaxBlobs)))  OutDataTypeStr=uint8
  Saturation : Saturate  UpperLimit=255  LowerLimit=0
  Switch : Switch  Criteria=u2 ~= 0  SaturateOnIntegerOverflow=off  InputSameDT=off
  bit2RGB : Subsystem
  Out1 : Outport  SampleTime=1.2796101795549e-07  VectorParamsAs1DForOutWhenUnconnected=off
  wires:
  1-D Lookup Table/1 -> Delay/1
  Add/1 -> Switch/1
  Constant/1 -> Add/2
  Delay/1 -> bit2RGB/1(In1)
  Gain1/1 -> Add/1
  Saturation/1 -> 1-D Lookup Table/1
  Switch/1 -> Saturation/1
  bit2RGB/1(Out1) -> Out1/1
  In1/1 -> Switch/3, Switch/2, Gain1/1

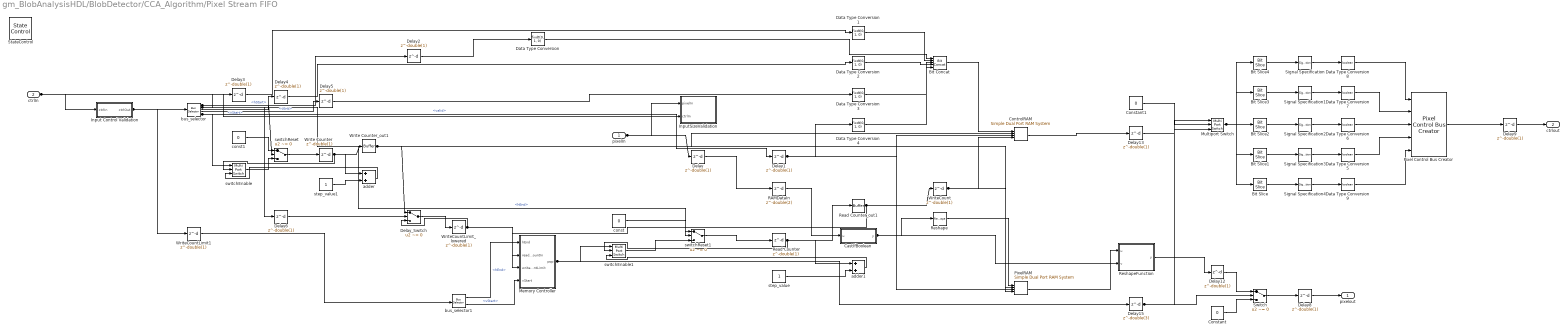
== system gm_BlobAnalysisHDL/BlobDetector/CCA_Algorithm/Pixel Stream FIFO ==
  pixelIn : Inport  OutDataTypeStr=fixdt(0,8,0,'DataTypeOverride', 'Off')  SampleTime=1.2796101795549e-07
  ctrlIn : Inport  Port=2  SampleTime=1.2796101795549e-07
  Bit Concat : hdlsllib/Logic and Bit Operations/Bit Concat  numInputs=5
  Bit Slice : hdlsllib/Logic and Bit Operations/Bit Slice  lidx=double(0)  ridx=double(0)
  Bit Slice1 : hdlsllib/Logic and Bit Operations/Bit Slice  lidx=double(1)  ridx=double(1)
  Bit Slice2 : hdlsllib/Logic and Bit Operations/Bit Slice  lidx=double(2)  ridx=double(2)
  Bit Slice3 : hdlsllib/Logic and Bit Operations/Bit Slice  lidx=double(3)  ridx=double(3)
  Bit Slice4 : hdlsllib/Logic and Bit Operations/Bit Slice  lidx=double(4)  ridx=double(4)
  CastIfBoolean : Subsystem
  Constant : Constant  Value=0  OutDataTypeStr=uint8  SampleTime=1.2796101795549e-07
  Constant1 : Constant  Value=0  OutDataTypeStr=fixdt(0, 5, 0)  SampleTime=1.2796101795549e-07
  ControlRAM : hdlsllib/HDL RAMs/Simple Dual Port RAM System  RAMType=Simple dual port  WriteOutputValue=New data  RAMInitialValue=0  SimulateUsing=Code generation
  Data Type Conversion{,1..4} (5 alike) : DataTypeConversion  OutDataTypeStr=fixdt(0, 1, 0)  SampleTime=1.2796101795549e-07  SaturateOnIntegerOverflow=off  RndMeth=Floor
  Data Type Conversion{5..9} (5 alike) : DataTypeConversion  OutDataTypeStr=boolean  SampleTime=1.2796101795549e-07  SaturateOnIntegerOverflow=off  RndMeth=Floor
  Delay{,1..6,8,12..13} (10 alike) : Delay  DelayLength=double(1)  InitialCondition=0  SampleTime=1.2796101795549e-07
  Delay15 : Delay  DelayLength=double(3)  InitialCondition=0  SampleTime=1.2796101795549e-07
  Delay9 : Delay  DelayLength=double(1)  SampleTime=1.2796101795549e-07
  Delay_Switch : Switch  Criteria=u2 ~= 0  Threshold=double(0)  OutDataTypeStr=fixdt(0, 11, 0)  SampleTime=1.2796101795549e-07  SaturateOnIntegerOverflow=off  InputSameDT=off
  "Input Control Validation " : Subsystem
  InputSizeValidation : Subsystem
  Memory Controller : Subsystem
  Multiport Switch : MultiPortSwitch  DataPortOrder=Zero-based contiguous  Inputs=2  DiagnosticForDefault=None  zeroidx=on  OutDataTypeStr=fixdt(0, 5, 0)  SampleTime=1.2796101795549e-07  SaturateOnIntegerOverflow=off  InputSameDT=off
  Pixel Control Bus Creator : visionhdlutilities/Pixel Control Bus Creator
  PixelRAM : hdlsllib/HDL RAMs/Simple Dual Port RAM System  RAMType=Simple dual port  WriteOutputValue=New data  RAMInitialValue=0  SimulateUsing=Code generation
  RAMDataIn : Delay  DelayLength=double(2)  InitialCondition=0  SampleTime=1.2796101795549e-07
  Read Counter : Delay  DelayLength=double(1)  InitialCondition=0  SampleTime=1.2796101795549e-07
  Read Counter_out1 : hdlmdlgenlib/Buffer
  Reshape : Reshape
  ReshapeFunction : Subsystem
  Signal Specification{,1..4} (5 alike) : SignalSpecification  OutDataTypeStr=fixdt(0, 1, 0)  Dimensions=1
  StateControl : StateControl  StateControl=Synchronous
  Switch : Switch  Criteria=u2 ~= 0  Threshold=double(0)  OutDataTypeStr=uint8  SampleTime=1.2796101795549e-07  SaturateOnIntegerOverflow=off  InputSameDT=off
  Write Counter : Delay  DelayLength=double(1)  InitialCondition=0  SampleTime=1.2796101795549e-07
  Write Counter_out1 : hdlmdlgenlib/Buffer
  WriteCount : Delay  DelayLength=double(1)  InitialCondition=0  SampleTime=1.2796101795549e-07
  WriteCountLimit1 : Delay  DelayLength=double(1)  SampleTime=1.2796101795549e-07
  WriteCountLimit_lowered : Delay  DelayLength=double(1)  InitialCondition=0  SampleTime=1.2796101795549e-07
  adder : Sum  AccumDataTypeStr=fixdt(0, 11, 0)  OutDataTypeStr=fixdt(0, 11, 0)  SampleTime=1.2796101795549e-07
  adder1 : Sum  AccumDataTypeStr=fixdt(0, 11, 0)  OutDataTypeStr=fixdt(0, 11, 0)  SampleTime=1.2796101795549e-07
  bus_selector : BusSelector  OutputSignals=hStart,hEnd,vStart,vEnd,valid
  bus_selector1 : BusSelector  OutputSignals=hEnd,vStart
  const : Constant  Value=0  VectorParams1D=off  OutDataTypeStr=fixdt(0, 11, 0)  SampleTime=1.2796101795549e-07
  const1 : Constant  Value=0  VectorParams1D=off  OutDataTypeStr=fixdt(0, 11, 0)  SampleTime=1.2796101795549e-07
  step_value : Constant  VectorParams1D=off  OutDataTypeStr=fixdt(0, 11, 0)  SampleTime=1.2796101795549e-07
  step_value1 : Constant  VectorParams1D=off  OutDataTypeStr=fixdt(0, 11, 0)  SampleTime=1.2796101795549e-07
  switchEnable : MultiPortSwitch  DataPortOrder=Zero-based contiguous  Inputs=2  DiagnosticForDefault=None  zeroidx=on  OutDataTypeStr=fixdt(0, 11, 0)  SampleTime=1.2796101795549e-07  SaturateOnIntegerOverflow=off  InputSameDT=off
  switchEnable1 : MultiPortSwitch  DataPortOrder=Zero-based contiguous  Inputs=2  DiagnosticForDefault=None  zeroidx=on  OutDataTypeStr=fixdt(0, 11, 0)  SampleTime=1.2796101795549e-07  SaturateOnIntegerOverflow=off  InputSameDT=off
  switchReset : Switch  Criteria=u2 ~= 0  Threshold=double(0)  OutDataTypeStr=fixdt(0, 11, 0)  SampleTime=1.2796101795549e-07  SaturateOnIntegerOverflow=off  InputSameDT=off
  switchReset1 : Switch  Criteria=u2 ~= 0  Threshold=double(0)  OutDataTypeStr=fixdt(0, 11, 0)  SampleTime=1.2796101795549e-07  SaturateOnIntegerOverflow=off  InputSameDT=off
  pixelout : Outport  SampleTime=1.2796101795549e-07
  ctrlout : Outport  Port=2  SampleTime=1.2796101795549e-07
  wires:
  Bit Concat/1 -> ControlRAM/1
  Bit Slice/1 -> Signal Specification4/1
  Bit Slice1/1 -> Signal Specification3/1
  Bit Slice2/1 -> Signal Specification2/1
  Bit Slice3/1 -> Signal Specification1/1
  Bit Slice4/1 -> Signal Specification/1
  CastIfBoolean/1(y) -> Reshape/1, ReshapeFunction/2(v)
  Constant/1 -> Switch/3
  Constant1/1 -> Multiport Switch/2
  ControlRAM/1 -> Delay13/1
  Data Type Conversion/1 -> Bit Concat/1
  Data Type Conversion1/1 -> Bit Concat/2
  Data Type Conversion2/1 -> Bit Concat/3
  Data Type Conversion3/1 -> Bit Concat/4
  Data Type Conversion4/1 -> Bit Concat/5
  Data Type Conversion5/1 -> Pixel Control Bus Creator/4
  Data Type Conversion6/1 -> Pixel Control Bus Creator/3
  Data Type Conversion7/1 -> Pixel Control Bus Creator/2
  Data Type Conversion8/1 -> Pixel Control Bus Creator/1
  Data Type Conversion9/1 -> Pixel Control Bus Creator/5
  Delay/1 -> RAMDataIn/1
  Delay1/1 -> Data Type Conversion4/1, PixelRAM/3, ControlRAM/3
  Delay12/1 -> Switch/1
  Delay13/1 -> Multiport Switch/3
  Delay15/1 -> Switch/2, Multiport Switch/1
  Delay2/1 -> Data Type Conversion/1
  Delay3/1 -> Data Type Conversion1/1
  Delay4/1 -> Data Type Conversion2/1
  Delay5/1 -> Data Type Conversion3/1
  Delay6/1 -> Delay_Switch/2
  Delay8/1 -> pixelout/1
  Delay9/1 -> ctrlout/1
  "Input Control Validation "/1(ctrlOut) -> bus_selector/1, WriteCountLimit1/1
  Memory Controller/1(pop) -> Delay15/1, switchEnable1/1
  Multiport Switch/1 -> Bit Slice4/1, Bit Slice3/1, Bit Slice2/1, Bit Slice1/1, Bit Slice/1
  Pixel Control Bus Creator/1 -> Delay9/1
  bus_selector/1 -> Delay2/1, switchReset/2  "<hStart>"
  bus_selector/2 -> Delay6/1, Delay3/1, switchReset1/2  "<hEnd>"
  bus_selector/3 -> Delay4/1  "<vStart>"
  bus_selector/4 -> Delay5/1  "<vEnd>"
  bus_selector/5 -> Delay1/1, switchEnable/1  "<valid>"
  bus_selector1/1 -> Memory Controller/1(hEnd)  "<hEnd>"
  bus_selector1/2 -> Memory Controller/4(vStart)  "<vStart>"
  PixelRAM/1 -> ReshapeFunction/1(u)
  RAMDataIn/1 -> CastIfBoolean/1(u)
  Read Counter_out1/1 -> WriteCount/1, Memory Controller/2(readCountIn)
  Reshape/1 -> PixelRAM/1
  ReshapeFunction/1(y) -> Delay12/1
  Signal Specification/1 -> Data Type Conversion8/1
  Signal Specification1/1 -> Data Type Conversion7/1
  Signal Specification2/1 -> Data Type Conversion6/1
  Signal Specification3/1 -> Data Type Conversion5/1
  Signal Specification4/1 -> Data Type Conversion9/1
  Switch/1 -> Delay8/1
  Write Counter_out1/1 -> Delay_Switch/1, PixelRAM/2, ControlRAM/2
  WriteCount/1 -> PixelRAM/4, ControlRAM/4
  WriteCountLimit_lowered/1 -> Memory Controller/3(writeCountLimit), Delay_Switch/3
  WriteCountLimit1/1 -> bus_selector1/1
  const/1 -> switchReset1/1
  step_value/1 -> adder1/2
  Write Counter/1 -> Write Counter_out1/1, switchEnable/2, adder/1
  const1/1 -> switchReset/1
  step_value1/1 -> adder/2
  pixelIn/1 -> Delay/1, InputSizeValidation/1(pixelIn)
  ctrlIn/1 -> "Input Control Validation "/1(ctrlIn), InputSizeValidation/2(ctrlIn)
  adder1/1 -> switchEnable1/3
  switchEnable1/1 -> switchReset1/3
  switchReset1/1 -> Read Counter/1
  Read Counter/1 -> Read Counter_out1/1, switchEnable1/2, adder1/1
  adder/1 -> switchEnable/3
  switchEnable/1 -> switchReset/3
  switchReset/1 -> Write Counter/1
  Delay_Switch/1 -> WriteCountLimit_lowered/1

== system gm_BlobAnalysisHDL/BlobDetector/CCA_Algorithm/TimingSubsystem ==
  Vid_i : Inport  OutDataTypeStr=boolean  PortDimensions=1  SampleTime=1.2796101795549e-07
  Ctrl_i : Inport  Port=2
  Pix_Pos : Subsystem
  create_rst : Subsystem
  Vid_o : Outport  SampleTime=1.2796101795549e-07  VectorParamsAs1DForOutWhenUnconnected=off
  Ctrl_o : Outport  Port=2  VectorParamsAs1DForOutWhenUnconnected=off
  Rst_o : Outport  Port=3  SampleTime=1.2796101795549e-07  VectorParamsAs1DForOutWhenUnconnected=off
  X : Outport  Port=4  SampleTime=1.2796101795549e-07  VectorParamsAs1DForOutWhenUnconnected=off
  Y : Outport  Port=5  SampleTime=1.2796101795549e-07  VectorParamsAs1DForOutWhenUnconnected=off
  wires:
  Pix_Pos/1(Column) -> X/1
  Pix_Pos/2(Row) -> Y/1
  create_rst/1(Video_o) -> Vid_o/1
  create_rst/2(Ctrl_o) -> Pix_Pos/1(Ctrl_i), Ctrl_o/1
  create_rst/3(Rst) -> Pix_Pos/2(Rst), Rst_o/1
  Vid_i/1 -> create_rst/1(Video_i)
  Ctrl_i/1 -> create_rst/2(ctrl_i)
